simulink model "HW04_DecouplingControl_stepchange"  (R2023b)
settings: Solver=VariableStepAuto  StartTime=0.0  StopTime=150  RelTol=1e-3
libraries: slpidlib x2
settings Model: Creator=ssjang  LastModifiedBy=YYlab_05
settings OptimizationCC: ReuseModelBlockBuffer=off

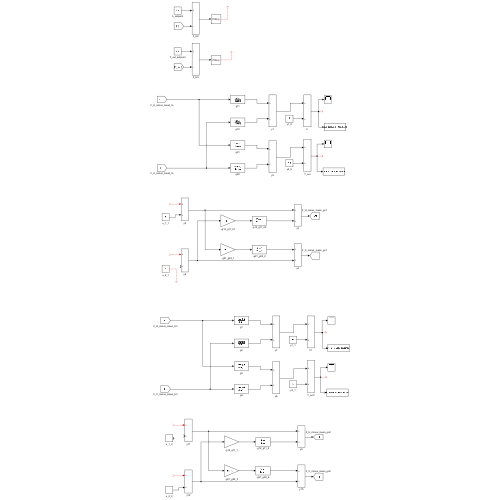
[thumbnail: Simulink's stored preview of the top-level diagram]
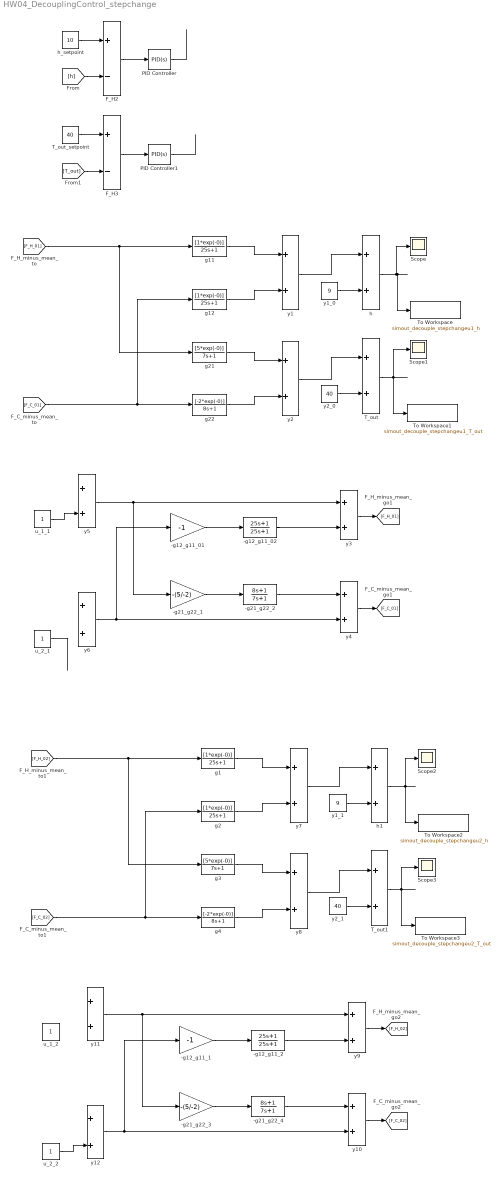
== system HW04_DecouplingControl_stepchange ==
  -g12_g11_01 : Gain  Gain=-1
  -g12_g11_02 : TransferFcn  Numerator=[25 1]  Denominator=[25 1]
  -g12_g11_1 : Gain  Gain=-1
  -g12_g11_2 : TransferFcn  Numerator=[25 1]  Denominator=[25 1]
  -g21_g22_1 : Gain  Gain=-(5/-2)
  -g21_g22_2 : TransferFcn  Numerator=[8 1]  Denominator=[7 1]
  -g21_g22_3 : Gain  Gain=-(5/-2)
  -g21_g22_4 : TransferFcn  Numerator=[8 1]  Denominator=[7 1]
  F_H2 : Sum  Inputs=+-
  F_H3 : Sum  Inputs=+-
  PID Controller : slpidlib/PID Controller  Controller=PID  Form=Parallel  TimeDomain=Continuous-time  UseExternalTs=off  SampleTime=-1  IntegratorMethod=Forward Euler  FilterMethod=Forward Euler  ControllerParametersSource=internal  P=0.102031913284982  I=0.012941042087745  UseKiTs=off  D=0.0340315618564053  N=15.1726685649185  UseFilter=on  TunerSelectOption=Transfer Function Based (PID Tuner App)  InitialConditionSource=internal  InitialConditionForIntegrator=0  InitialConditionForFilter=0  DifferentiatorICPrevScaledInput=0  ExternalReset=none  TrackingMode=off  Kt=1  LimitOutput=off  SatLimitsSource=internal  UpperSaturationLimit=inf  LowerSaturationLimit=-inf  LinearizeAsGain=on  AntiWindupMode=none  Kb=1  LimitIntegrator=off  UpperIntegratorSaturationLimit=inf  LowerIntegratorSaturationLimit=-inf  POutMin=[]  POutMax=[]  IOutMin=[]  IOutMax=[]  DOutMin=[]  DOutMax=[]  NOutMin=[]  NOutMax=[]  SumOutMin=[]  SumOutMax=[]  SaturationOutMin=[]  SaturationOutMax=[]  PParamMin=[]  PParamMax=[]  IParamMin=[]  IParamMax=[]  DParamMin=[]  DParamMax=[]  NParamMin=[]  NParamMax=[]  KbParamMin=[]  KbParamMax=[]  KtParamMin=[]  KtParamMax=[]  KbOutMin=[]  KbOutMax=[]  KtOutMin=[]  KtOutMax=[]  IntegratorOutMin=[]  IntegratorOutMax=[]  FilterOutMin=[]  FilterOutMax=[]  SumI1OutMin=[]  SumI1OutMax=[]  SumI2OutMin=[]  SumI2OutMax=[]  SumI3OutMin=[]  SumI3OutMax=[]  SumI4OutMin=[]  SumI4OutMax=[]  SumDOutMin=[]  SumDOutMax=[]  DifferentiatorOutMin=[]  DifferentiatorOutMax=[]  FilterDiffOutCoefMin=[]  FilterDiffOutCoefMax=[]  ReciprocalOutMin=[]  ReciprocalOutMax=[]  SumDenOutMin=[]  SumDenOutMax=[]  SumNumOutMin=[]  SumNumOutMax=[]  DivideOutMin=[]  DivideOutMax=[]  UdiffTsProdOutMin=[]  UdiffTsProdOutMax=[]  NTsProdOutMin=[]  NTsProdOutMax=[]  UintegralTsProdOutMin=[]  UintegralTsProdOutMax=[]  UngainTsProdOutMin=[]  UngainTsProdOutMax=[]  ClampingZeroOutDataTypeStr=Inherit: Inherit via back propagation  ClampingZeroOutMin=[]  ClampingZeroOutMax=[]  FilterDenConstantOutDataTypeStr=Inherit: Inherit via back propagation  FilterDenConstantOutMin=[]  FilterDenConstantOutMax=[]  PCopyOutDataTypeStr=Inherit: Inherit via back propagation  PCopyOutMin=[]  PCopyOutMax=[]  NCopyOutDataTypeStr=Inherit: Inherit via back propagation  NCopyOutMin=[]  NCopyOutMax=[]  IntegratorContinuousStateAttributes=''  IntegratorStateMustResolveToSignalObject=off  IntegratorRTWStateStorageClass=Auto  FilterContinuousStateAttributes=''  FilterStateMustResolveToSignalObject=off  FilterRTWStateStorageClass=Auto  ParallelPVariant=InternalParameters  IdealPVariant=Disabled  IVariant=InternalParameters  DVariant=InternalParameters  IntegratorVariant=Continuous  SatVariant=Disabled  AWVariant=Passthrough  PCopyVariant=Disabled  TRVariant=Disabled  FdbkBlocksVariant=Forward  IdealPFdbkVariant=Disabled  SatFdbkVariant=Disabled  DerivativeFilterVariant=ContFilter  NVariant=InternalParameters  NCopyVariant=Disabled  FilterICVariant=InternalICsFilter  IntegratorICVariant=InternalICs  ExternalResetVariant=Disabled  TRSumVariant=Passthrough  SumFdbkVariant=Disabled  SumVariant=Sum_PID  TsampFilterVariant=InternalTs  TsampNgainVariant=Passthrough  TsampIntegralVariant=Disabled_SignalSpec  ExternalSaturationOutDataTypeStr=Inherit: Same as second input
  PID Controller1 : slpidlib/PID Controller  Controller=PID  Form=Parallel  TimeDomain=Continuous-time  UseExternalTs=off  SampleTime=-1  IntegratorMethod=Forward Euler  FilterMethod=Forward Euler  ControllerParametersSource=internal  P=0  I=-1  UseKiTs=off  D=0  N=100  UseFilter=on  TunerSelectOption=Transfer Function Based (PID Tuner App)  InitialConditionSource=internal  InitialConditionForIntegrator=0  InitialConditionForFilter=0  DifferentiatorICPrevScaledInput=0  ExternalReset=none  TrackingMode=off  Kt=1  LimitOutput=off  SatLimitsSource=internal  UpperSaturationLimit=inf  LowerSaturationLimit=-inf  LinearizeAsGain=on  AntiWindupMode=none  Kb=1  LimitIntegrator=off  UpperIntegratorSaturationLimit=inf  LowerIntegratorSaturationLimit=-inf  POutMin=[]  POutMax=[]  IOutMin=[]  IOutMax=[]  DOutMin=[]  DOutMax=[]  NOutMin=[]  NOutMax=[]  SumOutMin=[]  SumOutMax=[]  SaturationOutMin=[]  SaturationOutMax=[]  PParamMin=[]  PParamMax=[]  IParamMin=[]  IParamMax=[]  DParamMin=[]  DParamMax=[]  NParamMin=[]  NParamMax=[]  KbParamMin=[]  KbParamMax=[]  KtParamMin=[]  KtParamMax=[]  KbOutMin=[]  KbOutMax=[]  KtOutMin=[]  KtOutMax=[]  IntegratorOutMin=[]  IntegratorOutMax=[]  FilterOutMin=[]  FilterOutMax=[]  SumI1OutMin=[]  SumI1OutMax=[]  SumI2OutMin=[]  SumI2OutMax=[]  SumI3OutMin=[]  SumI3OutMax=[]  SumI4OutMin=[]  SumI4OutMax=[]  SumDOutMin=[]  SumDOutMax=[]  DifferentiatorOutMin=[]  DifferentiatorOutMax=[]  FilterDiffOutCoefMin=[]  FilterDiffOutCoefMax=[]  ReciprocalOutMin=[]  ReciprocalOutMax=[]  SumDenOutMin=[]  SumDenOutMax=[]  SumNumOutMin=[]  SumNumOutMax=[]  DivideOutMin=[]  DivideOutMax=[]  UdiffTsProdOutMin=[]  UdiffTsProdOutMax=[]  NTsProdOutMin=[]  NTsProdOutMax=[]  UintegralTsProdOutMin=[]  UintegralTsProdOutMax=[]  UngainTsProdOutMin=[]  UngainTsProdOutMax=[]  ClampingZeroOutDataTypeStr=Inherit: Inherit via back propagation  ClampingZeroOutMin=[]  ClampingZeroOutMax=[]  FilterDenConstantOutDataTypeStr=Inherit: Inherit via back propagation  FilterDenConstantOutMin=[]  FilterDenConstantOutMax=[]  PCopyOutDataTypeStr=Inherit: Inherit via back propagation  PCopyOutMin=[]  PCopyOutMax=[]  NCopyOutDataTypeStr=Inherit: Inherit via back propagation  NCopyOutMin=[]  NCopyOutMax=[]  IntegratorContinuousStateAttributes=''  IntegratorStateMustResolveToSignalObject=off  IntegratorRTWStateStorageClass=Auto  FilterContinuousStateAttributes=''  FilterStateMustResolveToSignalObject=off  FilterRTWStateStorageClass=Auto  ParallelPVariant=InternalParameters  IdealPVariant=Disabled  IVariant=InternalParameters  DVariant=InternalParameters  IntegratorVariant=Continuous  SatVariant=Disabled  AWVariant=Passthrough  PCopyVariant=Disabled  TRVariant=Disabled  FdbkBlocksVariant=Forward  IdealPFdbkVariant=Disabled  SatFdbkVariant=Disabled  DerivativeFilterVariant=ContFilter  NVariant=InternalParameters  NCopyVariant=Disabled  FilterICVariant=InternalICsFilter  IntegratorICVariant=InternalICs  ExternalResetVariant=Disabled  TRSumVariant=Passthrough  SumFdbkVariant=Disabled  SumVariant=Sum_PID  TsampFilterVariant=InternalTs  TsampNgainVariant=Passthrough  TsampIntegralVariant=Disabled_SignalSpec  ExternalSaturationOutDataTypeStr=Inherit: Same as second input
  Scope{,1..3} (4 alike) : Scope
  T_out : Sum
  T_out1 : Sum
  T_out_setpoint : Constant  Value=40
  To Workspace : ToWorkspace  VariableName=simout_decouple_stepchangeu1_h  SaveFormat=Timeseries  SampleTime=-1
  To Workspace1 : ToWorkspace  VariableName=simout_decouple_stepchangeu1_T_out  SaveFormat=Timeseries  SampleTime=-1
  To Workspace2 : ToWorkspace  VariableName=simout_decouple_stepchangeu2_h  SaveFormat=Timeseries  SampleTime=-1
  To Workspace3 : ToWorkspace  VariableName=simout_decouple_stepchangeu2_T_out  SaveFormat=Timeseries  SampleTime=-1
  g{1..2,11..12} (4 alike) : TransferFcn  Numerator=[1*exp(-0)]  Denominator=[25 1]
  g21 : TransferFcn  Numerator=[5*exp(-0)]  Denominator=[7 1]
  g22 : TransferFcn  Numerator=[-2*exp(-0)]  Denominator=[8 1]
  g3 : TransferFcn  Numerator=[5*exp(-0)]  Denominator=[7 1]
  g4 : TransferFcn  Numerator=[-2*exp(-0)]  Denominator=[8 1]
  h : Sum
  h1 : Sum
  h_setpoint : Constant  Value=10
  u_1_1 : Constant
  u_1_2 : Constant
  u_2_1 : Constant
  u_2_2 : Constant
  y{1..12} (12 alike) : Sum
  y1_0 : Constant  Value=9
  y1_1 : Constant  Value=9
  y2_0 : Constant  Value=40
  y2_1 : Constant  Value=40
  wires:
  [F_H_01] -> g21/1, g11/1
  [F_C_01] -> g12/1, g22/1
  g11/1 -> y1/1
  g12/1 -> y1/2
  y1/1 -> h/1
  g22/1 -> y2/2
  g21/1 -> y2/1
  y2/1 -> T_out/1
  y1_0/1 -> h/2
  y2_0/1 -> T_out/2
  h/1 -> Scope/1, To Workspace/1
  h_setpoint/1 -> F_H2/1
  [h] -> F_H2/2
  F_H2/1 -> PID Controller/1
  PID Controller/1 -> ?
  [T_out] -> F_H3/2
  T_out_setpoint/1 -> F_H3/1
  F_H3/1 -> PID Controller1/1
  T_out/1 -> To Workspace1/1, Scope1/1
  PID Controller1/1 -> ?
  -g12_g11_01/1 -> -g12_g11_02/1
  -g21_g22_1/1 -> -g21_g22_2/1
  y3/1 -> [F_H_01]
  y4/1 -> [F_C_01]
  y5/1 -> -g21_g22_1/1, y3/1
  y6/1 -> y4/2, -g12_g11_01/1
  -g12_g11_02/1 -> y3/2
  -g21_g22_2/1 -> y4/1
  u_1_1/1 -> y5/2
  ? -> y5/1
  ? -> y6/1
  u_2_1/1 -> ?
  u_2_2/1 -> y12/2
  y10/1 -> [F_C_02]
  -g12_g11_2/1 -> y9/2
  y12/1 -> y10/2, -g12_g11_1/1
  ? -> y12/1
  ? -> y11/1
  -g12_g11_1/1 -> -g12_g11_2/1
  y11/1 -> -g21_g22_3/1, y9/1
  h1/1 -> Scope2/1, To Workspace2/1
  -g21_g22_4/1 -> y10/1
  T_out1/1 -> To Workspace3/1, Scope3/1
  g4/1 -> y8/2
  g1/1 -> y7/1
  -g21_g22_3/1 -> -g21_g22_4/1
  y8/1 -> T_out1/1
  [F_H_02] -> g3/1, g1/1
  y7/1 -> h1/1
  [F_C_02] -> g2/1, g4/1
  y9/1 -> [F_H_02]
  y1_1/1 -> h1/2
  y2_1/1 -> T_out1/2
  g2/1 -> y7/2
  g3/1 -> y8/1
